simulink library "Contact_Forces_Lib"  (R2017b)
settings: Solver=ode45  StartTime=0.0  StopTime=10.0  RelTol=1e-3  EnableMultiTasking=on
undefined symbols (not defined in the file or in its folder): b_contact, ball, cone, custom_param_1, custom_param_2, Extr_Data_Ring, k_contact, l_cone, length_cylinder, length_tube, mu_kinetic, mu_static, pen_exponent, pen_full_damp_F, rad_s_cone, radius_cylinder, radius_tube, v_thr, X, Y, Z
libraries: nesl_utility x182, sm_lib x103, Contact_Forces_Lib x67, simulink x17, fl_lib x1
(part 11 of 11)

== system Contact_Forces_Lib/3D/Sphere to Cone Force/Forces/Ff/Resolve Ff/Ff in ConB/FConB ==
  sinazm : Inport
  cosazm : Inport  Port=2
  FRing : Inport  Port=3
  FAxis : Inport  Port=4
  Divide{1..4} (4 alike) : Product  Inputs=**
  Gain : Gain  Gain=cosConeTh
  Gain1 : Gain  Gain=sinConeTh
  Gain2 : Gain  Gain=-1
  Gain3 : Gain  Gain=-1
  Gain4 : Gain  Gain=-1
  Sum : Sum
  Sum1 : Sum
  FxConB : Outport
  FyConB : Outport  Port=2
  FzConB : Outport  Port=3
  wires:
  Gain4/1 -> Sum1/1
  Divide1/1 -> Gain4/1
  Sum1/1 -> FxConB/1  "FxConB"
  Gain3/1 -> Sum1/2
  Divide4/1 -> Gain3/1
  Sum/1 -> FyConB/1  "FyConB"
  Gain2/1 -> Sum/2
  Divide3/1 -> Gain2/1
  Gain/1 -> Divide4/2, Divide3/2
  Gain1/1 -> FzConB/1  "FzConB"
  sinazm/1 -> Divide1/2, Divide3/1
  cosazm/1 -> Divide2/2, Divide4/1
  Divide2/1 -> Sum/1
  FRing/1 -> Divide1/1, Divide2/1
  FAxis/1 -> Gain/1, Gain1/1

== system Contact_Forces_Lib/3D/Sphere to Cone Force/Forces/Ff/Resolve Ff/Ff in ConB/Tx in B ==
  FyConB : Inport
  FzConB : Inport  Port=2
  sinazm : Inport  Port=3
  z : Inport  Port=4
  rConAxtoCP : Inport  Port=5
  rSphtoCP : Inport  Port=6
  Divide1 : Product  Inputs=***
  Divide{2..5} (4 alike) : Product  Inputs=**
  Gain : Gain  Gain=cosConeTh
  Gain1 : Gain  Gain=sinConeTh
  Gain2 : Gain  Gain=-1
  Gain3 : Gain  Gain=-1
  Sum : Sum
  Sum1 : Sum
  TxConB : Outport
  TxSph_B : Outport  Port=2
  wires:
  Gain2/1 -> Sum1/2
  Sum1/1 -> TxSph_B/1
  Gain3/1 -> Sum/2
  rConAxtoCP/1 -> Divide1/3
  sinazm/1 -> Divide1/1, Divide5/1
  Divide4/1 -> Gain2/1
  Divide3/1 -> Sum1/1
  FyConB/1 -> Divide4/2, Divide2/1
  Gain/1 -> Divide4/1
  Divide5/1 -> Divide3/2
  Gain1/1 -> Divide5/2
  Divide2/1 -> Gain3/1
  z/1 -> Divide2/2
  rSphtoCP/1 -> Gain/1, Gain1/1
  FzConB/1 -> Divide1/2, Divide3/1
  Divide1/1 -> Sum/1
  Sum/1 -> TxConB/1

== system Contact_Forces_Lib/3D/Sphere to Cone Force/Forces/Ff/Resolve Ff/Ff in ConB/Ty in B ==
  FxConB : Inport
  FzConB : Inport  Port=2
  cosazm : Inport  Port=3
  z : Inport  Port=4
  rConAxtoCP : Inport  Port=5
  rSphtoCP : Inport  Port=6
  Divide1 : Product  Inputs=***
  Divide2 : Product  Inputs=**
  Divide4 : Product  Inputs=***
  Divide5 : Product  Inputs=**
  Gain : Gain  Gain=cosConeTh
  Gain1 : Gain  Gain=sinConeTh
  Gain2 : Gain  Gain=-1
  Gain3 : Gain  Gain=-1
  Sum : Sum
  Sum1 : Sum
  TyConB : Outport
  TySph_B : Outport  Port=2
  wires:
  Gain/1 -> Divide5/2
  Gain3/1 -> Sum/1
  FzConB/1 -> Divide4/3, Divide1/1
  Sum/1 -> TyConB/1
  Divide1/1 -> Gain3/1
  FxConB/1 -> Divide5/1, Divide2/1
  rSphtoCP/1 -> Gain1/1, Gain/1
  z/1 -> Divide2/2
  Gain1/1 -> Divide4/1
  cosazm/1 -> Divide4/2, Divide1/2
  Divide4/1 -> Gain2/1
  Divide5/1 -> Sum1/1
  Gain2/1 -> Sum1/2
  Sum1/1 -> TySph_B/1
  rConAxtoCP/1 -> Divide1/3
  Divide2/1 -> Sum/2

== system Contact_Forces_Lib/3D/Sphere to Cone Force/Forces/Ff/Resolve Ff/Ff in ConB/Tz in B ==
  FxConB : Inport
  FyConB : Inport  Port=2
  sinazm : Inport  Port=3
  cosazm : Inport  Port=4
  rConAxtoCP : Inport  Port=5
  rSphtoCP : Inport  Port=6
  FRing : Inport  Port=7
  Divide2 : Product  Inputs=**
  Divide4 : Product  Inputs=***
  Divide5 : Product  Inputs=***
  Gain1 : Gain  Gain=sinConeTh
  Gain4 : Gain  Gain=-1
  Sum1 : Sum
  TzConB : Outport
  TzSph_B : Outport  Port=2
  wires:
  FRing/1 -> Divide2/2
  rConAxtoCP/1 -> Divide2/1
  sinazm/1 -> Divide5/2
  Sum1/1 -> TzSph_B/1
  Divide4/1 -> Sum1/2
  Gain4/1 -> Sum1/1
  cosazm/1 -> Divide4/2
  Gain1/1 -> Divide5/3, Divide4/1
  rSphtoCP/1 -> Gain1/1
  FxConB/1 -> Divide5/1
  Divide2/1 -> TzConB/1
  Divide5/1 -> Gain4/1
  FyConB/1 -> Divide4/3

== system Contact_Forces_Lib/3D/Sphere to Tube Force/Forces/Ff/Resolve Ff/Ff in TubB/Tx in B ==
  sinazm : Inport
  FyTubB : Inport  Port=2
  FzTubB : Inport  Port=3
  z : Inport  Port=4
  rCyltoCp : Inport  Port=5
  rSphtoCP : Inport  Port=6
  Divide{1..2,5..6} (4 alike) : Product  Inputs=**
  Sum : Sum
  TxTubB : Outport
  TxSph_B : Outport  Port=2
  wires:
  Sum/1 -> TxTubB/1
  Divide1/1 -> TxSph_B/1
  FyTubB/1 -> Divide6/1
  Divide5/1 -> Divide2/1, Divide1/2
  rSphtoCP/1 -> Divide1/1
  rCyltoCp/1 -> Divide2/2
  FzTubB/1 -> Divide5/1
  sinazm/1 -> Divide5/2
  z/1 -> Divide6/2
  Divide6/1 -> Sum/2
  Divide2/1 -> Sum/1

== system Contact_Forces_Lib/3D/Sphere to Tube Force/Forces/Ff/Resolve Ff/Ff in TubB/Ty in B ==
  cosazm : Inport
  FxTubB : Inport  Port=2
  FzTubB : Inport  Port=3
  z : Inport  Port=4
  rCyltoCp : Inport  Port=5
  rSphtoCP : Inport  Port=6
  Divide{1..2,5..6} (4 alike) : Product  Inputs=**
  Gain2 : Gain  Gain=-1
  Sum : Sum
  TyTubB : Outport
  TySph_B : Outport  Port=2
  wires:
  Sum/1 -> TyTubB/1
  Gain2/1 -> Divide5/1
  Divide2/1 -> Sum/1
  Divide6/1 -> Sum/2
  z/1 -> Divide6/2
  cosazm/1 -> Divide5/2
  FzTubB/1 -> Gain2/1
  rCyltoCp/1 -> Divide2/2
  rSphtoCP/1 -> Divide1/1
  Divide5/1 -> Divide2/1, Divide1/2
  FxTubB/1 -> Divide6/1
  Divide1/1 -> TySph_B/1

== system Contact_Forces_Lib/3D/Sphere to Tube Force/Forces/Ff/Resolve Ff/Ff in TubB/Tz in B ==
  FRing : Inport
  rTubToCP : Inport  Port=2
  rSphToCP : Inport  Port=3
  Divide7 : Product  Inputs=**
  Divide8 : Product  Inputs=**
  TzTubB : Outport
  TzSphB : Outport  Port=2
  wires:
  FRing/1 -> Divide8/1, Divide7/1
  rSphToCP/1 -> Divide7/2
  rTubToCP/1 -> Divide8/2
  Divide7/1 -> TzSphB/1
  Divide8/1 -> TzTubB/1  "TzTubB"

== system Contact_Forces_Lib/3D/Prototype/Cone in Ring Force/Point of Contact calc/Force Calc/Computing Force from nonzero penetration points/For Iterator Subsystem/Linear ==
  Pen : Inport
  Pen Vel : Inport  Port=2
  Abs : Abs  ZeroCross=off
  Gain1 : Gain  Gain=k_pen  Multiplication=Matrix(K*u)  SaturateOnIntegerOverflow=on  OutDataTypeStr=Inherit: Same as input  ParamDataTypeStr=Inherit: Same as input
  Gain2 : Gain  Gain=-b_penvel  Multiplication=Matrix(K*u)  SaturateOnIntegerOverflow=on  OutDataTypeStr=Inherit: Same as input  ParamDataTypeStr=Inherit: Same as input
  Product : Product  RndMeth=Zero
  Saturation : Saturate  UpperLimit=Inf  LowerLimit=0  ZeroCross=off
  Sign : Signum  ZeroCross=off
  Spr F : Outport
  Damp F : Outport  Port=2
  wires:
  Gain1/1 -> Spr F/1  "Stiffness_Force"
  Gain2/1 -> Product/2  "Damping_Force"
  Pen Vel/1 -> Saturation/1  "Pen Vel"
  Sign/1 -> Abs/1
  Product/1 -> Damp F/1  "Damping_Force"
  Abs/1 -> Product/1  "Damping_Force_Enable"
  Pen/1 -> Gain1/1, Sign/1  "Penetration"
  Saturation/1 -> Gain2/1

== system Contact_Forces_Lib/3D/Prototype/Cylinder In Ring Force/Point of Contact calc/Force Calc/Computing Force from nonzero penetration points/For Iterator Subsystem/Linear ==
  Pen : Inport
  Pen Vel : Inport  Port=2
  Abs : Abs  ZeroCross=off
  Gain1 : Gain  Gain=k_pen  Multiplication=Matrix(K*u)  SaturateOnIntegerOverflow=on  OutDataTypeStr=Inherit: Same as input  ParamDataTypeStr=Inherit: Same as input
  Gain2 : Gain  Gain=-b_penvel  Multiplication=Matrix(K*u)  SaturateOnIntegerOverflow=on  OutDataTypeStr=Inherit: Same as input  ParamDataTypeStr=Inherit: Same as input
  Product : Product  RndMeth=Zero
  Saturation : Saturate  UpperLimit=Inf  LowerLimit=0  ZeroCross=off
  Sign : Signum  ZeroCross=off
  Spr F : Outport
  Damp F : Outport  Port=2
  wires:
  Gain1/1 -> Spr F/1  "Stiffness_Force"
  Gain2/1 -> Product/2  "Damping_Force"
  Pen Vel/1 -> Saturation/1  "Pen Vel"
  Sign/1 -> Abs/1
  Product/1 -> Damp F/1  "Damping_Force"
  Abs/1 -> Product/1  "Damping_Force_Enable"
  Pen/1 -> Gain1/1, Sign/1  "Penetration"
  Saturation/1 -> Gain2/1

== system Contact_Forces_Lib/3D/Sphere to Cone Force/Forces/Ff/Relative vel at CP/Calculate vRelRing/Alternate Calculation Method/vCPinRingWx ==
  cosazm : Inport
  rSphtoCP sign : Inport  Port=2
  wx : Inport  Port=3
  Constant : Constant  Value=pi/2
  Constant1 : Constant  Value=sinConeTh
  Constant2 : Constant  Value=cosConeTh
  Gain : Gain  Gain=-1
  Math Function : Math  Operator=square  SaturateOnIntegerOverflow=on
  Math Function1 : Math  Operator=square  SaturateOnIntegerOverflow=on
  Product : Product  Inputs=4
  Product1 : Product  Inputs=3
  Product2 : Product
  Sqrt : Sqrt  SaturateOnIntegerOverflow=on
  Subtract : Sum  Inputs=+-
  Subtract1 : Sum
  Trigonometric Function : Trigonometry  Operator=cos
  Trigonometric Function1 : Trigonometry  Operator=atan2
  vCPinRingWx : Outport
  wires:
  Gain/1 -> vCPinRingWx/1
  wx/1 -> Product/1
  rSphtoCP sign/1 -> Product1/1, Product2/1
  Constant2/1 -> Product2/2
  Constant1/1 -> Product1/2
  Math Function1/1 -> Subtract1/1
  Math Function/1 -> Subtract1/2
  cosazm/1 -> Product/4, Product1/3
  Subtract1/1 -> Sqrt/1
  Sqrt/1 -> Product/2
  Product1/1 -> Trigonometric Function1/2, Math Function/1  "Rx"
  Product2/1 -> Trigonometric Function1/1, Math Function1/1  "Rz"
  Trigonometric Function1/1 -> Subtract/2
  Constant/1 -> Subtract/1
  Subtract/1 -> Trigonometric Function/1
  Trigonometric Function/1 -> Product/3
  Product/1 -> Gain/1

== system Contact_Forces_Lib/3D/Sphere to Cone Force/Forces/Ff/Relative vel at CP/Calculate vRelRing/Alternate Calculation Method/vCPinRingWy ==
  sinazm : Inport
  rSphtoCP sign : Inport  Port=2
  wy : Inport  Port=3
  Constant : Constant  Value=pi/2
  Constant1 : Constant  Value=sinConeTh
  Constant2 : Constant  Value=cosConeTh
  Gain : Gain  Gain=-1
  Math Function : Math  Operator=square  SaturateOnIntegerOverflow=on
  Math Function1 : Math  Operator=square  SaturateOnIntegerOverflow=on
  Product : Product  Inputs=4
  Product1 : Product  Inputs=3
  Product2 : Product
  Sqrt : Sqrt  SaturateOnIntegerOverflow=on
  Subtract : Sum  Inputs=+-
  Subtract1 : Sum
  Trigonometric Function : Trigonometry  Operator=cos
  Trigonometric Function1 : Trigonometry  Operator=atan2
  vCPinRingWy : Outport
  wires:
  Product/1 -> Gain/1
  Trigonometric Function/1 -> Product/3
  Subtract/1 -> Trigonometric Function/1
  Constant/1 -> Subtract/1
  Trigonometric Function1/1 -> Subtract/2
  Product2/1 -> Math Function1/1, Trigonometric Function1/1  "Rz"
  Product1/1 -> Math Function/1, Trigonometric Function1/2  "Rx"
  Sqrt/1 -> Product/2
  Subtract1/1 -> Sqrt/1
  sinazm/1 -> Product1/3, Product/4
  Math Function/1 -> Subtract1/2
  Math Function1/1 -> Subtract1/1
  Constant1/1 -> Product1/2
  Constant2/1 -> Product2/2
  rSphtoCP sign/1 -> Product2/1, Product1/1
  wy/1 -> Product/1
  Gain/1 -> vCPinRingWy/1

== matlab function Contact_Forces_Lib/3D/Prototype/Cylinder In Ring Force/Point of Contact calc/Force Calc/MAX_ML/MATLAB Function ==
  data: pen input; x input; y input; xc output; yc output; penc output; ind output
function [xc, yc, penc,ind] = fcn(pen, x, y)
%#codegen
[val,ind] = max(pen);

% if val == 0
%     penc = 0;
%     xc = 0;
%     yc = 0; 
% else
    penc = pen(ind);
    xc = x(ind);
    yc = y(ind);
% end

== matlab function Contact_Forces_Lib/3D/Prototype/Cone in Ring Force/Point of Contact calc/Force Calc/MAX_ML/MATLAB Function ==
  data: pen input; x input; y input; xc output; yc output; penc output; ind output
function [xc, yc, penc,ind] = fcn(pen, x, y)
%#codegen
[val,ind] = max(pen);

% if val == 0
%     penc = 0;
%     xc = 0;
%     yc = 0; 
% else
    penc = pen(ind);
    xc = x(ind);
    yc = y(ind);
% end
